simulink model "AutoboxModel"  (R2019b)
settings: Solver=ode1  StartTime=0.0  StopTime=inf  FixedStep=0.01  RelTol=1e-3
PostLoadFcn:
  | , if any(exist('dsrtsu_mdlpostloadfcn', 'file') ~= 0), dsrtsu_mdlpostloadfcn('Execute', bdroot); end,
undefined symbols (not defined in the file or in its folder): Activation, Cancel, Clearance
libraries: simulink x4, Lib_Controller x2, Lib_CanCommunication x1, Lib_EthernetCommunication x1
settings Model: RTICANMMDATA=struct('GeneralSetupData',struct('modelroot','C:\Users\kessler\Documents\fav\apollo_opensource\modules\autobox_control','generalsettings',struct('filesettings',struct('destfolder',struct('Name','RTICANMM_FILES','Check',1),'buildfolder',struct('Name','.','Check',1),'AbsDestfolder',struct('Name','C:\Users\kessler\Documents\fav\apollo_opensource\modules\autobox_control\RTICANMM_FILES'),'AbsBuildfolder',struct('Name','C:\Users\kessler\Documents\fav\apollo_opensource\modules\autobox_control'))),'options',struct('addpaths',1,'rmpaths',1,'addtrcexclusion',true,'cannavigator',struct('checkmonitoring',0),'show_usrtrc',0,'use_usrtrc',0),'advanced',struct('options',ones(1,100)),'MPSetup',{{}},'RTI',struct('Type','RTI1401','Ver','7.13','Date','02-Nov-2019'),'modelname','AutoboxModel','block','AutoboxModel'))  DSRTSU_INTERNAL_RTIFPGA=150  DevelopmentMode=FunctionDevelopment  OptimizingMode=Automatic  DSRTSU_INTERNAL_RTI_VER=550  DSRTSU_INTERNAL_RTI_TYPE=rti1401  Creator=kessler  LastModifiedBy=kessler
settings DataIOCC: LimitDataPoints=on  SaveFormat=Array  SaveOutput=off  DSMLogging=off  SaveTime=off  ReturnWorkspaceOutputs=off
settings OptimizationCC: BlockReduction=off  BooleanDataType=off  OptimizeBlockIOStorage=off  BufferReuse=off  GlobalBufferReuse=off  ExpressionFolding=off  PassReuseOutputArgsThreshold=0  LocalBlockOutputs=off  OptimizeDataStoreBuffers=off  BusAssignmentInplaceUpdate=off
settings DebuggingCC: SaveWithParameterizedLinksMsg=none  SignalResolutionControl=TryResolveAllWithWarning  MultiTaskDSMMsg=warning  MultiTaskCondExecSysMsg=none  ParameterTunabilityLossMsg=error  SFUnexpectedBacktrackingDiag=warning  SFNoUnconditionalDefaultTransitionDiag=warning  SFExecutionAtInitializationDiag=none  ArithmeticOperatorsInVariantConditions=warning
settings HardwareCC: ProdBitPerPointer=32  ProdBitPerSizeT=32  ProdBitPerPtrDiffT=32  ProdLargestAtomicInteger=Integer  ProdEndianess=BigEndian  ProdWordSize=32  ProdHWDeviceType=Custom Processor->Custom  TargetBitPerPointer=64  TargetLongLongMode=on  TargetIntDivRoundTo=Zero  TargetEndianess=BigEndian  TargetHWDeviceType=Custom Processor->Custom
settings ModelReferenceCC: PropagateSignalLabelsOutOfModel=off
settings SFSimCC: SimUseLocalCustomCode=off  MATLABDynamicMemAlloc=off  CustomCodeUndefinedFunction=UseInterfaceOnly
settings RTWCC: Description=dSPACE DS1401 Hardware Platform  SystemTargetFile=rti1401.tlc  MakeCommand=make_rti  TemplateMakefile=rti1401.tmf  RTWVerbose=off  RTWUseLocalCustomCode=off
settings CodeAppCC: ForceParamTrailComments=on  OperatorAnnotations=on
settings STFCustomTargetCC: ParMdlRefBuildCompliant=on  SystemTargetFile=rti1401.tlc
settings GRTTargetCC: TargetLangStandard=C89/C90 (ANSI)  CompOptLevelCompliant=off  ConcurrentExecutionCompliant=off  CombineOutputUpdateFcns=off  MatFileLogging=off  CPPClassGenCompliant=off  UseToolchainInfoCompliant=off
settings ConfigComp: CovMetricSettings=dw  CovHtmlReporting=on  CovSaveCumulativeToWorkspaceVar=on  CovSaveSingleToWorkspaceVar=on  CovExternalEMLEnable=off

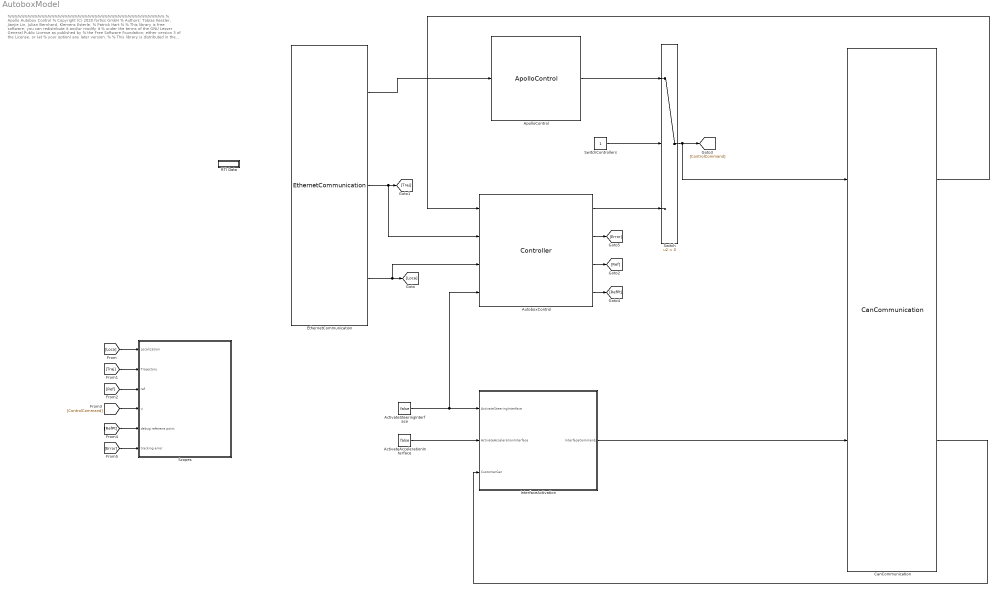
== system AutoboxModel ==
  note: %%%%%%%%%%%%%%%%%%%%%%%%%%%%%%%%%%%%%%%%%%%%%%%
      | % Apollo Autobox Control
      | % Copyright (C) 2020 fortiss GmbH
      | % Authors: Tobias Kessler, Jianjie Lin, Julian Bernhard, Klemens Esterle,
      | % Patrick Hart
      | %
      | % This library is free software; you can redistribute it and/or modify it
      | % under the terms of the GNU Lesser General Public License as published by
      | % the Free Software Foundation; either version 3 of the License, or (at
      | % your option) any later version.
      | %
      | % This library is distributed in the hope that it will be useful, but
      | % WITHOUT ANY WARRANTY; without even the implied warranty of
      | % MERCHANTABILITY or FITNESS FOR A PARTICULAR PURPOSE. See the GNU Lesser
      | % General Public License for more details.
      | %
      | % You should have received a copy of the GNU Lesser General Public License
      | % along with this library; if not, write to the Free Software Foundation,
      | % Inc., 51 Franklin Street, Fifth Floor, Boston, MA 02110-1301, USA.
      | %%%%%%%%%%%%%%%%%%%%%%%%%%%%%%%%%%%%%%%%%%%%%%%
  ActivateAccelerationInterface : Constant  Value=false  OutDataTypeStr=boolean
  ActivateSteeringInterface : Constant  Value=false  OutDataTypeStr=boolean
  ApolloControl : Lib_Controller/ApolloControl  SystemSampleTime=-1  Latency=0  AutoFrameSizeCalculation=off
  AutoboxControl : Lib_Controller/Controller  SystemSampleTime=-1  Latency=0  AutoFrameSizeCalculation=off
  CanCommunication : Lib_CanCommunication/CanCommunication  SystemSampleTime=-1  Latency=0  AutoFrameSizeCalculation=off
  EthernetCommunication : Lib_EthernetCommunication/EthernetCommunication  SystemSampleTime=-1  Latency=0  AutoFrameSizeCalculation=off
  InterfaceActivation : Subsystem
  RTI Data : Subsystem  Tag=struct('RTIDataServer',struct('RTIDataServerVs','2','RTIModelDescription','struct(''main'',''AutoboxModel'',''sub'',''AutoboxModel'',''isMp'',0)'))  LoadFcn="if exist('rtidc'), try,  rtidc('DataHostBlockClbLoad', gcbh); catch, disp(['Warning: ''LoadFcn'' for RTI Data block failed: ' lasterr]); end, end,"  mask(RTI_DATA_HOST){}
      mask help:
      | RTI Data Block.
      | This block is used by RTI to store internal model-dependent data.
      | Please keep this block on the root level of the model. Deleting this block will result in data loss.
      |
      | NEVER DELETE OR COPY THIS BLOCK!
      settings: CopyFcn="if exist('rtidc'), try,  rtidc('DataHostBlockClbCopy', gcbh); catch, disp(['Warning: ''CopyFcn'' for RTI Data block failed: ' lasterr]); end, end,"  DeleteFcn="if exist('rtidc'), try,  rtidc('DataHostBlockClbDelete', gcbh); catch, disp(['Warning: ''DeleteFcn'' for RTI Data block failed: ' lasterr]); end, end,"  ModelCloseFcn="if exist('rtidc'), try,  rtidc('DataHostBlockClbModelClose', gcbh); catch, disp(['Warning: ''ModelCloseFcn'' for RTI Data block failed: ' lasterr]); end, end,"  PreSaveFcn="if exist('rtidc'), try,  rtidc('DataHostBlockClbPreSave', gcbh); catch, disp(['Warning: ''PreSaveFcn'' for RTI Data block failed: ' lasterr]); end, end,"  PostSaveFcn="if exist('rtidc'), try,  rtidc('DataHostBlockClbPostSave', gcbh); catch, disp(['Warning: ''PostSaveFcn'' for RTI Data block failed: ' lasterr]); end, end,"  NameChangeFcn="if exist('rtidc'), try,  rtidc('DataHostBlockClbNameChange', gcbh); catch, disp(['Warning: ''NameChangeFcn'' for RTI Data block failed: ' lasterr]); end, end,"
      mask Help:
      | RTI Data Block.
      | This block is used by RTI to store internal model-dependent data.
      | Please keep this block on the root level of the model. Deleting this block will result in data loss.
      | 
      | NEVER DELETE OR COPY THIS BLOCK!
      mask Display: text(0.5, 0.5, 'RTI Data', 'HorizontalAlignment', 'center');
  Scopes : Subsystem
  Switch : Switch  Criteria=u2 > Threshold
  SwitchControllers : Constant
  wires:
  CanCommunication/2 -> InterfaceActivation/3(CustomerCan)
  Switch/1 -> CanCommunication/1, [ControlCommand]
  CanCommunication/1 -> AutoboxControl/1
  EthernetCommunication/2 -> AutoboxControl/2, [Traj]
  EthernetCommunication/3 -> [Loca], AutoboxControl/3
  ActivateSteeringInterface/1 -> AutoboxControl/4, InterfaceActivation/1(ActivateSteeringInterface)
  InterfaceActivation/1(InterfaceCommands) -> CanCommunication/2
  AutoboxControl/1 -> Switch/3
  EthernetCommunication/1 -> ApolloControl/1
  ApolloControl/1 -> Switch/1
  SwitchControllers/1 -> Switch/2
  ActivateAccelerationInterface/1 -> InterfaceActivation/2(ActivateAccelerationInterface)
  [Loca] -> Scopes/1(Localization)
  [Traj] -> Scopes/2(Trajectory)
  AutoboxControl/3 -> [Ref]
  [Ref] -> Scopes/3(ref)
  [ControlCommand] -> Scopes/4(u)
  AutoboxControl/4 -> [RefPt]
  [RefPt] -> Scopes/5(debug referene point)
  AutoboxControl/2 -> [Error]
  [Error] -> Scopes/6(tracking error)

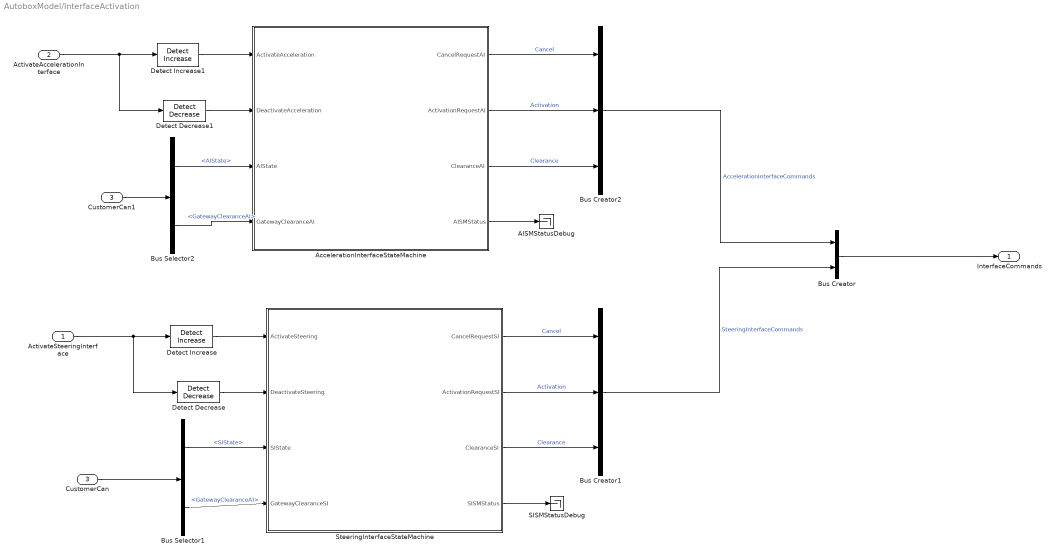
== system AutoboxModel/InterfaceActivation ==
  ActivateSteeringInterface : Inport
  ActivateAccelerationInterface : Inport  Port=2
  CustomerCan : Inport  Port=3
  AISMStatusDebug : Terminator
  AccelerationInterfaceStateMachine : Stateflow chart  TreatAsAtomicUnit=on
  Bus Creator : BusCreator  Inputs=2  OutDataTypeStr=Bus: InterfaceCommands  NonVirtualBus=on
  Bus Creator1 : BusCreator  Inputs=Cancel,Activation,Clearance  OutDataTypeStr=Bus: SteeringInterfaceCommands  NonVirtualBus=on
  Bus Creator2 : BusCreator  Inputs=Cancel,Activation,Clearance  OutDataTypeStr=Bus: AccelerationInterfaceCommands  NonVirtualBus=on
  Bus Selector1 : BusSelector  OutputSignals=Gateway_States.SIState,Gateway_States.GatewayClearanceAI
  Bus Selector2 : BusSelector  OutputSignals=Gateway_States.AIState,Gateway_States.GatewayClearanceAI
  CustomerCan1 : InportShadow  Port=3
  Detect Decrease : simulink/Logic and Bit Operations/Detect Decrease  vinit=0.0  OutDataTypeStr=boolean
  Detect Decrease1 : simulink/Logic and Bit Operations/Detect Decrease  vinit=0.0  OutDataTypeStr=boolean
  Detect Increase : simulink/Logic and Bit Operations/Detect Increase  vinit=0.0  OutDataTypeStr=boolean
  Detect Increase1 : simulink/Logic and Bit Operations/Detect Increase  vinit=0.0  OutDataTypeStr=boolean
  SISMStatusDebug : Terminator
  SteeringInterfaceStateMachine : Stateflow chart  TreatAsAtomicUnit=on
  InterfaceCommands : Outport  VectorParamsAs1DForOutWhenUnconnected=off
  wires:
  SteeringInterfaceStateMachine/2(ActivationRequestSI) -> Bus Creator1/2  "Activation"
  Bus Selector1/1 -> SteeringInterfaceStateMachine/3(SIState)  "<SIState>"
  ActivateSteeringInterface/1 -> Detect Decrease/1, Detect Increase/1
  CustomerCan/1 -> Bus Selector1/1
  Bus Creator/1 -> InterfaceCommands/1
  SteeringInterfaceStateMachine/3(ClearanceSI) -> Bus Creator1/3  "Clearance"
  SteeringInterfaceStateMachine/1(CancelRequestSI) -> Bus Creator1/1  "Cancel"
  Bus Selector1/2 -> SteeringInterfaceStateMachine/4(GatewayClearanceSI)  "<GatewayClearanceAI>"
  AccelerationInterfaceStateMachine/1(CancelRequestAI) -> Bus Creator2/1  "Cancel"
  AccelerationInterfaceStateMachine/2(ActivationRequestAI) -> Bus Creator2/2  "Activation"
  AccelerationInterfaceStateMachine/3(ClearanceAI) -> Bus Creator2/3  "Clearance"
  Bus Creator1/1 -> Bus Creator/2  "SteeringInterfaceCommands"
  Bus Creator2/1 -> Bus Creator/1  "AccelerationInterfaceCommands"
  Detect Increase/1 -> SteeringInterfaceStateMachine/1(ActivateSteering)
  Detect Decrease/1 -> SteeringInterfaceStateMachine/2(DeactivateSteering)
  SteeringInterfaceStateMachine/4(SISMStatus) -> SISMStatusDebug/1
  ActivateAccelerationInterface/1 -> Detect Decrease1/1, Detect Increase1/1
  Detect Increase1/1 -> AccelerationInterfaceStateMachine/1(ActivateAcceleration)
  Detect Decrease1/1 -> AccelerationInterfaceStateMachine/2(DeactivateAcceleration)
  CustomerCan1/1 -> Bus Selector2/1
  Bus Selector2/1 -> AccelerationInterfaceStateMachine/3(AIState)  "<AIState>"
  Bus Selector2/2 -> AccelerationInterfaceStateMachine/4(GatewayClearanceAI)  "<GatewayClearanceAI>"
  AccelerationInterfaceStateMachine/4(AISMStatus) -> AISMStatusDebug/1

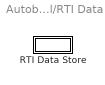
== system AutoboxModel/RTI Data ==
  RTI Data Store : Subsystem  Tag="struct('private',struct('version',struct('dsVer',uint32(2),'dsVerCreation',uint32(2),'RTI',struct('ver','7.4','type','RTI1401')),'access',struct('type','Model','isPerm',1,'created',['17-May-2018 12:59:00'],'modified',['29-Jun-2018 11:16:11'],'location','')),'public',struct('main',struct('data',[]),'sub',struct('name',{{'AutoboxModel'}},'data',{{struct('TH',struct('thTaskInfo',struct('taskType',{'TIMER','HWINT','TMRINT','SWINT','GLINT'},'tasksNumOf',{2,0,0,0,0},'srcIds',{{'TIMERA','TIMERA2'},{},{},{},{}},'taskNames',{{['Timer Task 1'],['Timer Task 2']},{},{},{},{}})),'th_tc',struct('dataType',{'TASK','TASK'},'taskGroupId',{'',''},'taskGroupList',{{},{}},'taskSchedulingPolicy',{'FCFS','FCFS'},'taskType',{'TIMER','TIMER'},'blkh',{-1,-1},'srcId',{'TIMERA','TIMERA2'},'srcSgnName',{['Timer A interrupt'],['Timer Task 1']},'srcCpuName',{'',''},'taskName',{['Timer Task 1  [0.01] s'],['Timer Task 2  [1] s']},'taskNameDisplayExt',{'',''},'smplTime',{0.01,1},'smplTimeOffs',{0,0},'hasFixedPriority',{0,0},'priority',{1,2},'hasFixedOvc',{0,0},'ovcType',{1,1},'ovcMax',{1,1}),'tc_th',struct('dataType',{'TASK','TASK'},'taskGroupId',{'',''},'taskGroupList',{{},{}},'taskSchedulingPolicy',{'FCFS','FCFS'},'taskType',{'TIMER','TIMER'},'blkh',{-1,-1},'srcId',{'TIMERA','TIMERA2'},'srcSgnName',{['Timer A interrupt'],['Timer Task 1']},'srcCpuName',{'',''},'taskName',{['Timer Task 1  [0.01] s'],['Timer Task 2  [1] s']},'taskNameDisplayExt',{'',''},'smplTime',{0.01,1},'smplTimeOffs',{0,0},'hasFixedPriority',{0,0},'priority',{1,2},'hasFixedOvc',{0,0},'ovcType',{1,1},'ovcMax',{1,1}))}})))"

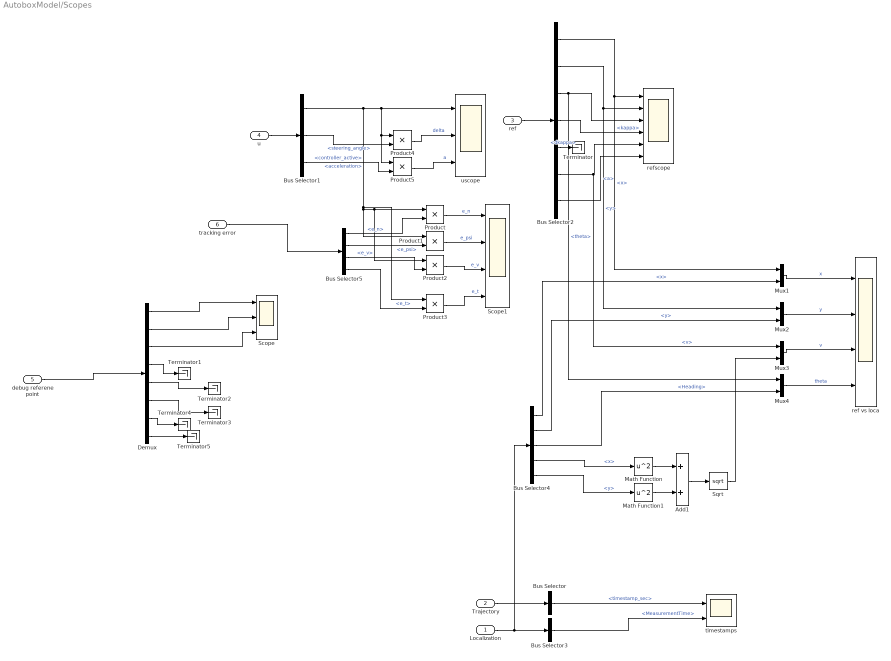
== system AutoboxModel/Scopes ==
  Localization : Inport  OutDataTypeStr=Bus: LocalizationToAutobox  BusOutputAsStruct=on
  Trajectory : Inport  Port=2  OutDataTypeStr=Bus: ControlTrajectory  BusOutputAsStruct=on
  ref : Inport  Port=3
  u : Inport  Port=4
  debug referene point : Inport  Port=5
  tracking error : Inport  Port=6
  Add1 : Sum
  Bus Selector : BusSelector  OutputSignals=timestamp_sec
  Bus Selector1 : BusSelector  OutputSignals=controller_active,steering_angle,acceleration
  Bus Selector2 : BusSelector  OutputSignals=x,y,theta,kappa,dkappa,v,a
  Bus Selector3 : BusSelector  OutputSignals=MeasurementTime
  Bus Selector4 : BusSelector  OutputSignals=Pose.Position.x,Pose.Position.y,Pose.Heading,Pose.LinearVelocity.x,Pose.LinearVelocity.y
  Bus Selector5 : BusSelector  OutputSignals=e_n,e_psi,e_v,e_t
  Demux : Demux  Outputs=8
  Math Function : Math  Operator=square  SaturateOnIntegerOverflow=on
  Math Function1 : Math  Operator=square  SaturateOnIntegerOverflow=on
  Mux{1..4} (4 alike) : Mux  Inputs=2
  Product{,1..5} (6 alike) : Product
  Scope : Scope  NumInputPorts=3
  Scope1 : Scope  NumInputPorts=4
  Sqrt : Sqrt  SaturateOnIntegerOverflow=on
  Terminator{,1..5} (6 alike) : Terminator
  ref vs loca : Scope  NumInputPorts=4
  refscope : Scope  NumInputPorts=6
  timestamps : Scope  NumInputPorts=2
  uscope : Scope  NumInputPorts=3
  wires:
  Bus Selector1/1 -> Product3/1, Product2/1, Product/1, Product1/1, Product5/1, Product4/1, uscope/1  "<controller_active>"
  Bus Selector1/2 -> Product4/2  "<steering_angle>"
  Bus Selector1/3 -> Product5/2  "<acceleration>"
  Bus Selector2/5 -> Terminator/1  "<dkappa>"
  u/1 -> Bus Selector1/1
  ref/1 -> Bus Selector2/1
  Bus Selector2/4 -> refscope/4  "<kappa>"
  Bus Selector2/3 -> Mux4/1, refscope/3  "<theta>"
  Bus Selector2/1 -> Mux1/1, refscope/1  "<x>"
  Bus Selector2/6 -> Mux3/1, refscope/5  "<v>"
  Bus Selector2/7 -> refscope/6  "<a>"
  Bus Selector2/2 -> Mux2/1, refscope/2  "<y>"
  Trajectory/1 -> Bus Selector/1
  Localization/1 -> Bus Selector4/1, Bus Selector3/1
  Bus Selector3/1 -> timestamps/2  "<MeasurementTime>"
  Bus Selector/1 -> timestamps/1  "<timestamp_sec>"
  Mux4/1 -> ref vs loca/4  "theta"
  Mux2/1 -> ref vs loca/2  "y"
  Mux3/1 -> ref vs loca/3  "v"
  Mux1/1 -> ref vs loca/1  "x"
  Bus Selector4/1 -> Mux1/2  "<x>"
  Bus Selector4/2 -> Mux2/2  "<y>"
  Bus Selector4/3 -> Mux4/2  "<Heading>"
  Math Function1/1 -> Add1/2
  Math Function/1 -> Add1/1
  Add1/1 -> Sqrt/1
  Bus Selector4/4 -> Math Function/1  "<x>"
  Bus Selector4/5 -> Math Function1/1  "<y>"
  Sqrt/1 -> Mux3/2
  Demux/3 -> Scope/3
  Demux/1 -> Scope/1
  Demux/2 -> Scope/2
  debug referene point/1 -> Demux/1
  Bus Selector5/2 -> Product1/2  "<e_psi>"
  Bus Selector5/4 -> Product3/2  "<e_t>"
  Bus Selector5/3 -> Product2/2  "<e_v>"
  Bus Selector5/1 -> Product/2  "<e_n>"
  tracking error/1 -> Bus Selector5/1
  Demux/4 -> Terminator1/1
  Demux/5 -> Terminator2/1
  Demux/6 -> Terminator3/1
  Demux/7 -> Terminator4/1
  Demux/8 -> Terminator5/1
  Product/1 -> Scope1/1  "e_n"
  Product1/1 -> Scope1/2  "e_psi"
  Product2/1 -> Scope1/3  "e_v"
  Product3/1 -> Scope1/4  "e_t"
  Product4/1 -> uscope/2  "delta"
  Product5/1 -> uscope/3  "a"

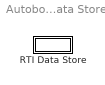
== system AutoboxModel/RTI Data/RTI Data Store ==
  RTI Data Store : Subsystem

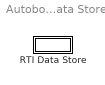
== system AutoboxModel/RTI Data/RTI Data Store/RTI Data Store ==
  RTI Data Store : Subsystem

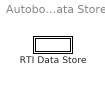
== system AutoboxModel/RTI Data/RTI Data Store/RTI Data Store/RTI Data Store ==
  RTI Data Store : Subsystem

== system AutoboxModel/RTI Data/RTI Data Store/RTI Data Store/RTI Data Store/RTI Data Store ==

== stateflow chart AutoboxModel/InterfaceActivation/AccelerationInterfaceStateMachine ==
  state Inactive
    entry: ClearanceAI=0;
    entry:CancelRequestAI=true;
    entry: AISMStatus=0;
  note: % AISMStatus könnte noch ein enum werden...
  state ActivationSequence
    state CheckAllPreconditions
      entry: AISMStatus=1;
    state PreconditionsSet
      entry: ClearanceAI=1;
      entry: AISMStatus=2;
    state SetCancelFalse
      entry: CancelRequestAI=false;
      entry: AISMStatus=3;
    state GatewayClearanceOk
      entry: ActivationRequestAI = true;
      exit: ActivationRequestAI = false;
      entry: AISMStatus=4;
    CheckAllPreconditions -> PreconditionsSet : [AIState==1] % door, seatbeld, gear
    PreconditionsSet -> SetCancelFalse : [GatewayClearanceAI==1] % gateway awaits activation
    SetCancelFalse -> GatewayClearanceOk : after(0.1,sec)
  state ActiveAcceleationControl
    entry: AISMStatus=5;
  (default) -> Inactive
  ActiveAcceleationControl -> Inactive [order 1] : [AIState~=2] % Gateway wirft ab
  ActiveAcceleationControl -> Inactive [order 2] : [DeactivateAcceleration] % Nutzer wirft ab
  Inactive -> CheckAllPreconditions : [ActivateAcceleration] % maybe && AIState==1 oder ~=13,14 hier?
  ActivationSequence -> Inactive : [DeactivateAcceleration]
  GatewayClearanceOk -> ActiveAcceleationControl : [AIState==2] % angle control
  data: ActivateAcceleration input boolean; DeactivateAcceleration input boolean; AIState input uint8; GatewayClearanceAI input boolean; CancelRequestAI output boolean; ActivationRequestAI output boolean; ClearanceAI output boolean; AISMStatus output uint8; data local double

== stateflow chart AutoboxModel/InterfaceActivation/SteeringInterfaceStateMachine ==
  state Inactive
    entry: ClearanceSI=0;
    entry:CancelRequestSI=true;
    entry: SISMStatus=0;
  note: % SISMStatus könnte noch ein enum werden...
  state ActivationSequence
    state CheckAllPreconditions
      entry: SISMStatus=1;
    state PreconditionsSet
      entry: ClearanceSI=1; %steering angle control
      entry: SISMStatus=2;
    state SetCancelFalse
      entry: CancelRequestSI=false;
      entry: SISMStatus=3;
    state GatewayClearanceOk
      entry: ActivationRequestSI = true;
      exit: ActivationRequestSI = false;
      entry: SISMStatus=4;
    CheckAllPreconditions -> PreconditionsSet : [SIState==1] % door, seatbeld, gear
    PreconditionsSet -> SetCancelFalse : [GatewayClearanceSI==1] % gateway awaits activation
    SetCancelFalse -> GatewayClearanceOk : after(0.1,sec)
  state ActiveSteeringAngleControl
    entry: SISMStatus=5;
  (default) -> Inactive
  ActiveSteeringAngleControl -> Inactive [order 1] : [SIState~=2] % Gatewa wirft ab
  ActiveSteeringAngleControl -> Inactive [order 2] : [DeactivateSteering] % Nutzer wirft ab
  Inactive -> CheckAllPreconditions : [ActivateSteering] % maybe && SIState==1 oder ~=13,14 hier?
  ActivationSequence -> Inactive : [DeactivateSteering]
  GatewayClearanceOk -> ActiveSteeringAngleControl : [SIState==2] % angle control
  data: ActivateSteering input boolean; DeactivateSteering input boolean; SIState input uint8; GatewayClearanceSI input boolean; CancelRequestSI output boolean; ActivationRequestSI output boolean; ClearanceSI output uint8; SISMStatus output uint8
